simulink model "controllermodel"  (R2020a)
settings: Solver=FixedStepDiscrete  StartTime=0.0  StopTime=10.0  FixedStep=1/100  RelTol=1e-3
undefined symbols (not defined in the file): DiscIntNeverNeededParam
libraries: simulink_extras x3
settings Model: Creator=janik  LastModifiedBy=hopfj
settings OptimizationCC: DefaultParameterBehavior=Inlined  EnhancedBackFolding=on  PassReuseOutputArgsAs=Individual arguments  ZeroExternalMemoryAtStartup=off  ZeroInternalMemoryAtStartup=off  OptimizeBlockOrder=speed  DifferentSizesBufferReuse=on  OptimizationCustomize=off  EfficientTunableParamExpr=on
settings DebuggingCC: ParameterTunabilityLossMsg=error
settings SFSimCC: MATLABDynamicMemAlloc=off
settings RTWCC: SystemTargetFile=ert.tlc  GenCodeOnly=on  TemplateMakefile=ert_default_tmf  GenerateReport=on  Toolchain=Microsoft Visual C++ 2019 v16.0 | nmake (64-bit Windows)  LaunchReport=on  TargetLang=C++
settings CodeAppCC: ForceParamTrailComments=on  IgnoreCustomStorageClasses=off  OperatorAnnotations=on  SimulinkDataObjDesc=on  SFDataObjDesc=on  MATLABFcnDesc=on  InsertBlockDesc=on
settings ERTTargetCC: TargetLangStandard=C++03 (ISO)  GenerateSampleERTMain=on  CodeInterfacePackaging=C++ class  SupportVariableSizeSignals=on  InlinedParameterPlacement=NonHierarchical  RootIOFormat=Structure reference  ERTCustomFileTemplate=example_file_process.tlc

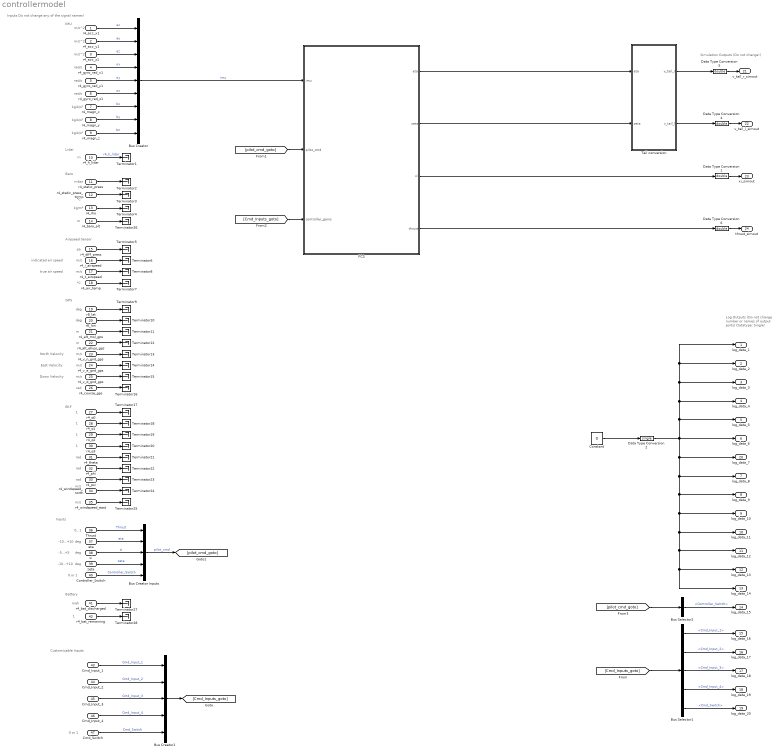
== system controllermodel ==
  note: Simulation Outputs
      | (Do not change!)
  note: m/s
  note: m/s
  note: Lidar
  note: kg/A/s²
  note: m/s
  note: m/s^2
  note: 1
  note: rad
  note: Down Velocity
  note: m
  note: m/s
  note: East Velocity
  note: kg/A/s²
  note: Inputs
      | Do not change any of the
      | signal names!
  note: m/s
  note: rad/s
  note: Airpseed Sensor
  note: Baro
  note: °C
  note: m/s
  note: Customizable Inputs
  note: kg/m³
  note: IMU
  note: pa
  note: 0...1
  note: m/s^2
  note: rad/s
  note: rad
  note: true air speed
  note: North Velocity
  note: mah
  note: m
  note: GPS
  note: kg/A/s²
  note: m/s
  note: rad/s
  note: mbar
  note: rad
  note: Inputs
  note: indicated air speed
  note: °C
  note: m
  note: m
  note: rad
  note: EKF
  note: Battery
  note: deg
  note: m/s^2
  note: deg
  note: Log Outputs
      | (Do not change
      | number or names
      | of output ports)
      | Datatype: Single!
  note: 0 or 1
  note: deg
  note: deg
  note: deg
  note: 1
  note: 1
  note: 1
  note: 1
  note: -10...+10
  note: -5...+5
  note: -10...+10
  note: 0 or 1
  r4_acc_x1 : Inport  OutDataTypeStr=single  Unit=m/s^2  PortDimensions=1  SampleTime=1/100  Interpolate=off
  r4_acc_y1 : Inport  Port=2  OutDataTypeStr=single  Unit=m/s^2  PortDimensions=1  SampleTime=1/100  Interpolate=off
  r4_acc_z1 : Inport  Port=3  OutDataTypeStr=single  Unit=m/s^2  PortDimensions=1  SampleTime=1/100  Interpolate=off
  r4_gyro_rad_x1 : Inport  Port=4  OutDataTypeStr=single  Unit=rad/s  PortDimensions=1  SampleTime=1/100  Interpolate=off
  r4_gyro_rad_y1 : Inport  Port=5  OutDataTypeStr=single  Unit=rad/s  PortDimensions=1  SampleTime=1/100  Interpolate=off
  r4_gyro_rad_z1 : Inport  Port=6  OutDataTypeStr=single  Unit=rad/s  PortDimensions=1  SampleTime=1/100  Interpolate=off  LockScale=on
  r4_magn_x : Inport  Port=7  OutDataTypeStr=single  Unit=kg/A/s^2  PortDimensions=1  SampleTime=1/100  Interpolate=off
  r4_magn_y : Inport  Port=8  OutDataTypeStr=single  Unit=kg/A/s^2  PortDimensions=1  SampleTime=1/100  Interpolate=off
  r4_magn_z : Inport  Port=9  OutDataTypeStr=single  Unit=kg/A/s^2  PortDimensions=1  SampleTime=1/100  Interpolate=off
  r4_h_lidar : Inport  Port=10  OutDataTypeStr=single  Unit=m  PortDimensions=1  SampleTime=1/100  Interpolate=off
  r4_static_press : Inport  Port=11  OutDataTypeStr=single  Unit=mbar  PortDimensions=1  SampleTime=1/100  Interpolate=off
  r4_static_press_temp : Inport  Port=12  OutDataTypeStr=single  Unit=°C  PortDimensions=1  SampleTime=1/100  Interpolate=off
  r4_rho : Inport  Port=13  OutDataTypeStr=single  Unit=kg/m^3  PortDimensions=1  SampleTime=1/100  Interpolate=off
  r4_baro_alt : Inport  Port=14  OutDataTypeStr=single  Unit=m  PortDimensions=1  SampleTime=1/100  Interpolate=off
  r4_diff_press : Inport  Port=15  OutDataTypeStr=single  Unit=Pa  PortDimensions=1  SampleTime=1/100  Interpolate=off
  r4_i_airspeed : Inport  Port=16  OutDataTypeStr=single  Unit=m/s  PortDimensions=1  SampleTime=1/100  Interpolate=off
  r4_t_airspeed : Inport  Port=17  OutDataTypeStr=single  Unit=m/s  PortDimensions=1  SampleTime=1/100  Interpolate=off
  r4_air_temp : Inport  Port=18  OutDataTypeStr=single  Unit=°C  PortDimensions=1  SampleTime=1/100  Interpolate=off
  r8_lat : Inport  Port=19  OutDataTypeStr=double  Unit=deg  PortDimensions=1  SampleTime=1/100  Interpolate=off
  r8_lon : Inport  Port=20  OutDataTypeStr=double  Unit=deg  PortDimensions=1  SampleTime=1/100  Interpolate=off
  r4_alt_msl_gps : Inport  Port=21  OutDataTypeStr=single  Unit=m  PortDimensions=1  SampleTime=1/100  Interpolate=off
  r4_alt_ellips_gps : Inport  Port=22  OutDataTypeStr=single  Unit=m  PortDimensions=1  SampleTime=1/100  Interpolate=off
  r4_v_n_gnd_gps : Inport  Port=23  OutDataTypeStr=single  Unit=m/s  PortDimensions=1  SampleTime=1/100  Interpolate=off
  r4_v_e_gnd_gps : Inport  Port=24  OutDataTypeStr=single  Unit=m/s  PortDimensions=1  SampleTime=1/100  Interpolate=off
  r4_v_d_gnd_gps : Inport  Port=25  OutDataTypeStr=single  Unit=m/s  PortDimensions=1  SampleTime=1/100  Interpolate=off
  r4_course_gps : Inport  Port=26  OutDataTypeStr=single  Unit=rad  PortDimensions=1  SampleTime=1/100  Interpolate=off
  r4_q0 : Inport  Port=27  OutMin=[-1]  OutMax=[1]  OutDataTypeStr=single  Unit=1  PortDimensions=1  SampleTime=1/100  Interpolate=off
  r4_q1 : Inport  Port=28  OutMin=[-1]  OutMax=[1]  OutDataTypeStr=single  Unit=1  PortDimensions=1  SampleTime=1/100  Interpolate=off
  r4_q2 : Inport  Port=29  OutMin=[-1]  OutMax=[1]  OutDataTypeStr=single  Unit=1  PortDimensions=1  SampleTime=1/100  Interpolate=off
  r4_q3 : Inport  Port=30  OutMin=[-1]  OutMax=[1]  OutDataTypeStr=single  Unit=one  PortDimensions=1  SampleTime=1/100  Interpolate=off
  r4_theta : Inport  Port=31  OutDataTypeStr=single  Unit=rad  PortDimensions=1  SampleTime=1/100  Interpolate=off
  r4_phi : Inport  Port=32  OutDataTypeStr=single  Unit=rad  PortDimensions=1  SampleTime=1/100  Interpolate=off
  r4_psi : Inport  Port=33  OutDataTypeStr=single  Unit=rad  PortDimensions=1  SampleTime=1/100  Interpolate=off
  r4_windspeed_north : Inport  Port=34  OutDataTypeStr=single  Unit=m/s  PortDimensions=1  SampleTime=1/100  Interpolate=off
  r4_windspeed_east : Inport  Port=35  OutDataTypeStr=single  Unit=m/s  PortDimensions=1  SampleTime=1/100  Interpolate=off
  Thrust : Inport  Port=36  OutDataTypeStr=single  PortDimensions=1  SampleTime=1/100  Interpolate=off
  eta : Inport  Port=37  OutDataTypeStr=single  Unit=deg  PortDimensions=1  SampleTime=1/100  Interpolate=off
  xi : Inport  Port=38  OutDataTypeStr=single  Unit=deg  PortDimensions=1  SampleTime=1/100  Interpolate=off
  zeta : Inport  Port=39  OutDataTypeStr=single  Unit=deg  PortDimensions=1  SampleTime=1/100  Interpolate=off
  Controller_Switch : Inport  Port=40  OutDataTypeStr=single  PortDimensions=1  SampleTime=1/100  Interpolate=off
  r4_bat_discharged : Inport  Port=41  OutDataTypeStr=single  Unit=mA*hr  PortDimensions=1  SampleTime=1/100  Interpolate=off
  r4_bat_remaining : Inport  Port=42  OutDataTypeStr=single  PortDimensions=1  SampleTime=1/100  Interpolate=off
  Cmd_Input_1 : Inport  Port=43  OutDataTypeStr=single  PortDimensions=1  SampleTime=1/100  Interpolate=off
  Cmd_Input_2 : Inport  Port=44  OutDataTypeStr=single  PortDimensions=1  SampleTime=1/100  Interpolate=off
  Cmd_Input_3 : Inport  Port=45  OutDataTypeStr=single  PortDimensions=1  SampleTime=1/100  Interpolate=off
  Cmd_Input_4 : Inport  Port=46  OutDataTypeStr=single  PortDimensions=1  SampleTime=1/100  Interpolate=off
  Cmd_Switch : Inport  Port=47  OutDataTypeStr=single  PortDimensions=1  SampleTime=1/100  Interpolate=off
  Bus Creator : BusCreator  Inputs=9
  Bus Creator Inputs : BusCreator  Inputs=5
  Bus Creator1 : BusCreator  Inputs=5
  Bus Selector1 : BusSelector  OutputSignals=Cmd_Input_1,Cmd_Input_2,Cmd_Input_3,Cmd_Input_4,Cmd_Switch
  Bus Selector2 : BusSelector  OutputSignals=Controller_Switch
  Constant : Constant  Value=0
  Data Type Conversion{1,4..6} (4 alike) : DataTypeConversion  OutDataTypeStr=double  RndMeth=Nearest
  Data Type Conversion2 : DataTypeConversion  OutDataTypeStr=single  RndMeth=Nearest
  FCS : Subsystem
  Tail conversion : Subsystem
  Terminator{1..28} (28 alike) : Terminator
  log_data_1 : Outport  OutDataTypeStr=single  SampleTime=1/100  VectorParamsAs1DForOutWhenUnconnected=off
  log_data_2 : Outport  Port=2  OutDataTypeStr=single  SampleTime=1/100  VectorParamsAs1DForOutWhenUnconnected=off
  log_data_3 : Outport  Port=3  OutDataTypeStr=single  SampleTime=1/100  VectorParamsAs1DForOutWhenUnconnected=off
  log_data_4 : Outport  Port=4  OutDataTypeStr=single  SampleTime=1/100  VectorParamsAs1DForOutWhenUnconnected=off
  log_data_5 : Outport  Port=5  OutDataTypeStr=single  SampleTime=1/100  VectorParamsAs1DForOutWhenUnconnected=off
  log_data_6 : Outport  Port=6  OutDataTypeStr=single  SampleTime=1/100  VectorParamsAs1DForOutWhenUnconnected=off
  log_data_8 : Outport  Port=7  OutDataTypeStr=single  SampleTime=1/100  VectorParamsAs1DForOutWhenUnconnected=off
  log_data_9 : Outport  Port=8  OutDataTypeStr=single  SampleTime=1/100  VectorParamsAs1DForOutWhenUnconnected=off
  log_data_10 : Outport  Port=9  OutDataTypeStr=single  SampleTime=1/100  VectorParamsAs1DForOutWhenUnconnected=off
  log_data_11 : Outport  Port=10  OutDataTypeStr=single  SampleTime=1/100  VectorParamsAs1DForOutWhenUnconnected=off
  log_data_12 : Outport  Port=11  OutDataTypeStr=single  SampleTime=1/100  VectorParamsAs1DForOutWhenUnconnected=off
  log_data_13 : Outport  Port=12  OutDataTypeStr=single  SampleTime=1/100  VectorParamsAs1DForOutWhenUnconnected=off
  log_data_14 : Outport  Port=13  OutDataTypeStr=single  SampleTime=1/100  VectorParamsAs1DForOutWhenUnconnected=off
  log_data_15 : Outport  Port=14  OutDataTypeStr=single  SampleTime=1/100  VectorParamsAs1DForOutWhenUnconnected=off
  log_data_16 : Outport  Port=15  OutDataTypeStr=single  SampleTime=1/100  VectorParamsAs1DForOutWhenUnconnected=off
  log_data_17 : Outport  Port=16  OutDataTypeStr=single  SampleTime=1/100  VectorParamsAs1DForOutWhenUnconnected=off
  log_data_18 : Outport  Port=17  OutDataTypeStr=single  SampleTime=1/100  VectorParamsAs1DForOutWhenUnconnected=off
  log_data_19 : Outport  Port=18  OutDataTypeStr=single  SampleTime=1/100  VectorParamsAs1DForOutWhenUnconnected=off
  log_data_20 : Outport  Port=19  OutDataTypeStr=single  SampleTime=1/100  VectorParamsAs1DForOutWhenUnconnected=off
  log_data_7 : Outport  Port=20  OutDataTypeStr=single  SampleTime=1/100  VectorParamsAs1DForOutWhenUnconnected=off
  v_tail_r_simout : Outport  Port=21  OutDataTypeStr=double  Unit=rad  SampleTime=1/100  VectorParamsAs1DForOutWhenUnconnected=off
  v_tail_l_simout : Outport  Port=22  OutDataTypeStr=double  Unit=rad  SampleTime=1/100  VectorParamsAs1DForOutWhenUnconnected=off
  xi_simout : Outport  Port=23  OutDataTypeStr=double  Unit=rad  SampleTime=1/100  VectorParamsAs1DForOutWhenUnconnected=off
  thrust_simout : Outport  Port=24  OutDataTypeStr=double  SampleTime=1/100  VectorParamsAs1DForOutWhenUnconnected=off
  wires:
  r4_phi/1 -> Terminator22/1
  Controller_Switch/1 -> Bus Creator Inputs/5  "Controller_Switch"
  r4_h_lidar/1 -> Terminator1/1  "r4_h_lidar"
  r4_gyro_rad_y1/1 -> Bus Creator/5  "oy"
  r4_rho/1 -> Terminator4/1
  FCS/1(eta) -> Tail conversion/1(eta)
  r4_static_press_temp/1 -> Terminator3/1
  r4_air_temp/1 -> Terminator7/1
  r4_alt_msl_gps/1 -> Terminator11/1
  r4_diff_press/1 -> Terminator5/1
  r4_acc_z1/1 -> Bus Creator/3  "az"
  xi/1 -> Bus Creator Inputs/3  "xi"
  Thrust/1 -> Bus Creator Inputs/1  "Thrust"
  r4_course_gps/1 -> Terminator16/1
  r4_q0/1 -> Terminator17/1
  Tail conversion/1(v_tail_r) -> Data Type Conversion5/1
  r4_v_n_gnd_gps/1 -> Terminator13/1
  Tail conversion/2(v_tail_l) -> Data Type Conversion4/1
  r4_magn_x/1 -> Bus Creator/7  "bx"
  FCS/3(xi) -> Data Type Conversion1/1
  r4_acc_y1/1 -> Bus Creator/2  "ay"
  r4_psi/1 -> Terminator23/1
  r4_v_e_gnd_gps/1 -> Terminator14/1
  r4_gyro_rad_x1/1 -> Bus Creator/4  "ox"
  r4_bat_discharged/1 -> Terminator27/1
  r4_baro_alt/1 -> Terminator26/1
  FCS/4(thrust) -> Data Type Conversion6/1
  r4_v_d_gnd_gps/1 -> Terminator15/1
  r4_q2/1 -> Terminator19/1
  r4_static_press/1 -> Terminator2/1
  Cmd_Input_1/1 -> Bus Creator1/1  "Cmd_Input_1"
  r4_gyro_rad_z1/1 -> Bus Creator/6  "oz"
  zeta/1 -> Bus Creator Inputs/4  "zeta"
  r4_magn_z/1 -> Bus Creator/9  "bz"
  r8_lat/1 -> Terminator9/1
  r8_lon/1 -> Terminator10/1
  r4_t_airspeed/1 -> Terminator8/1
  r4_magn_y/1 -> Bus Creator/8  "by"
  Cmd_Input_2/1 -> Bus Creator1/2  "Cmd_Input_2"
  r4_alt_ellips_gps/1 -> Terminator12/1
  r4_windspeed_east/1 -> Terminator25/1
  r4_windspeed_north/1 -> Terminator24/1
  Cmd_Input_4/1 -> Bus Creator1/4  "Cmd_Input_4"
  FCS/2(zeta) -> Tail conversion/2(zeta)
  eta/1 -> Bus Creator Inputs/2  "eta"
  Cmd_Input_3/1 -> Bus Creator1/3  "Cmd_Input_3"
  r4_q1/1 -> Terminator18/1
  r4_q3/1 -> Terminator20/1
  r4_bat_remaining/1 -> Terminator28/1
  r4_i_airspeed/1 -> Terminator6/1
  r4_acc_x1/1 -> Bus Creator/1  "ax"
  Constant/1 -> Data Type Conversion2/1
  Bus Creator/1 -> FCS/1(imu)  "imu"
  r4_theta/1 -> Terminator21/1
  Bus Creator1/1 -> [Cmd_Inputs_goto]
  [Cmd_Inputs_goto] -> Bus Selector1/1
  Bus Creator Inputs/1 -> [pilot_cmd_goto]  "pilot_cmd"
  Data Type Conversion1/1 -> xi_simout/1
  Data Type Conversion5/1 -> v_tail_r_simout/1
  Data Type Conversion4/1 -> v_tail_l_simout/1
  Data Type Conversion6/1 -> thrust_simout/1
  [pilot_cmd_goto] -> FCS/2(pilot_cmd)
  [Cmd_Inputs_goto] -> FCS/3(controller_gains)
  Data Type Conversion2/1 -> log_data_1/1, log_data_2/1, log_data_3/1, log_data_4/1, log_data_5/1, log_data_6/1, log_data_7/1, log_data_8/1, log_data_9/1, log_data_10/1, log_data_11/1, log_data_14/1, log_data_13/1, log_data_12/1
  Bus Selector1/2 -> log_data_17/1  "<Cmd_Input_2>"
  Bus Selector1/3 -> log_data_18/1  "<Cmd_Input_3>"
  Bus Selector1/4 -> log_data_19/1  "<Cmd_Input_4>"
  Bus Selector1/5 -> log_data_20/1  "<Cmd_Switch>"
  [pilot_cmd_goto] -> Bus Selector2/1
  Bus Selector2/1 -> log_data_15/1  "<Controller_Switch>"
  Cmd_Switch/1 -> Bus Creator1/5  "Cmd_Switch"
  Bus Selector1/1 -> log_data_16/1  "<Cmd_Input_1>"

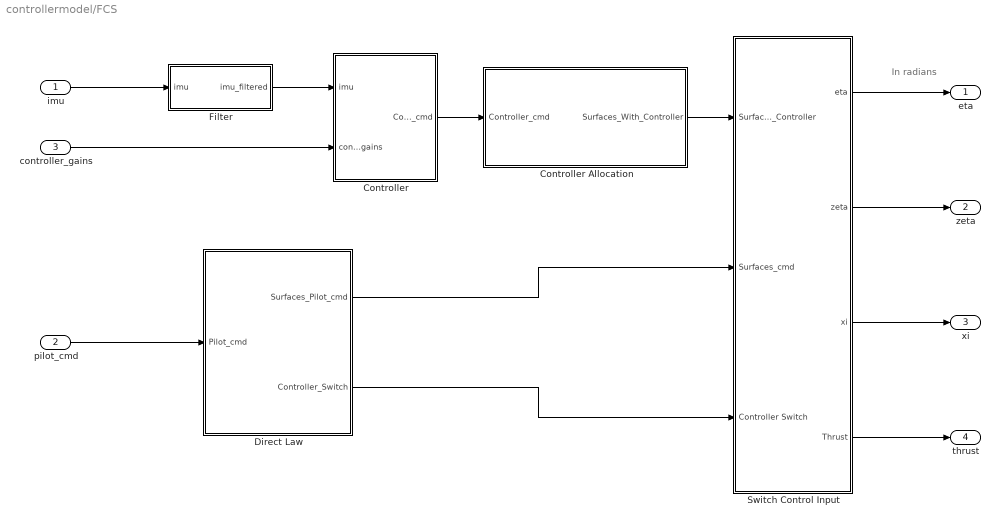
== system controllermodel/FCS ==
  note: In radians
  imu : Inport
  pilot_cmd : Inport  Port=2
  controller_gains : Inport  Port=3
  Controller : Subsystem
  Controller Allocation : Subsystem
  Direct Law : Subsystem
  Filter : Subsystem
  Switch Control Input : Subsystem
  eta : Outport  Unit=rad
  zeta : Outport  Port=2  Unit=rad
  xi : Outport  Port=3  Unit=rad
  thrust : Outport  Port=4  Unit=rad
  wires:
  Controller Allocation/1(Surfaces_With_Controller) -> Switch Control Input/1(Surfaces_With_Controller)
  pilot_cmd/1 -> Direct Law/1(Pilot_cmd)
  imu/1 -> Filter/1(imu)
  Switch Control Input/4(Thrust) -> thrust/1
  Switch Control Input/2(zeta) -> zeta/1
  Switch Control Input/1(eta) -> eta/1
  Switch Control Input/3(xi) -> xi/1
  Filter/1(imu_filtered) -> Controller/1(imu)
  Direct Law/2(Controller_Switch) -> Switch Control Input/3(Controller Switch)
  controller_gains/1 -> Controller/2(controller_gains)
  Direct Law/1(Surfaces_Pilot_cmd) -> Switch Control Input/2(Surfaces_cmd)
  Controller/1(Controller_cmd) -> Controller Allocation/1(Controller_cmd)

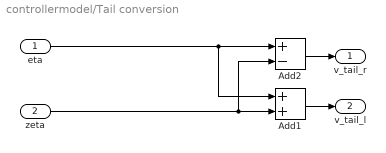
== system controllermodel/Tail conversion ==
  eta : Inport  Unit=rad
  zeta : Inport  Port=2  Unit=rad
  Add1 : Sum  OutDataTypeStr=double
  Add2 : Sum  Inputs=+-  InputSameDT=on  OutDataTypeStr=double
  v_tail_r : Outport  Unit=rad
  v_tail_l : Outport  Port=2  Unit=rad
  wires:
  Add1/1 -> v_tail_l/1
  Add2/1 -> v_tail_r/1
  zeta/1 -> Add2/2, Add1/2
  eta/1 -> Add2/1, Add1/1

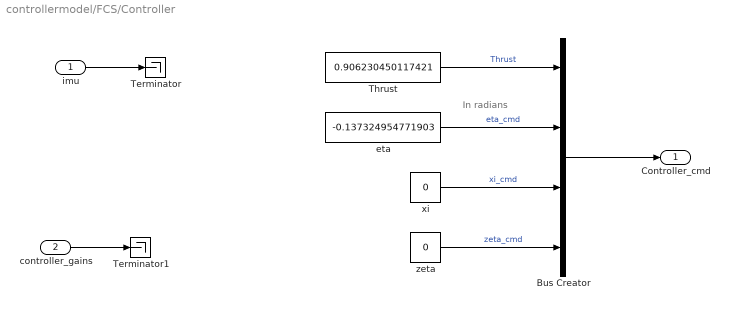
== system controllermodel/FCS/Controller ==
  note: In radians
  imu : Inport
  controller_gains : Inport  Port=2
  Bus Creator : BusCreator  Inputs=4
  Terminator : Terminator
  Terminator1 : Terminator
  Thrust : Constant  Value=0.906230450117421
  eta : Constant  Value=-0.137324954771903
  xi : Constant  Value=0
  zeta : Constant  Value=0
  Controller_cmd : Outport
  wires:
  Bus Creator/1 -> Controller_cmd/1
  imu/1 -> Terminator/1
  controller_gains/1 -> Terminator1/1
  Thrust/1 -> Bus Creator/1  "Thrust"
  eta/1 -> Bus Creator/2  "eta_cmd"
  xi/1 -> Bus Creator/3  "xi_cmd"
  zeta/1 -> Bus Creator/4  "zeta_cmd"

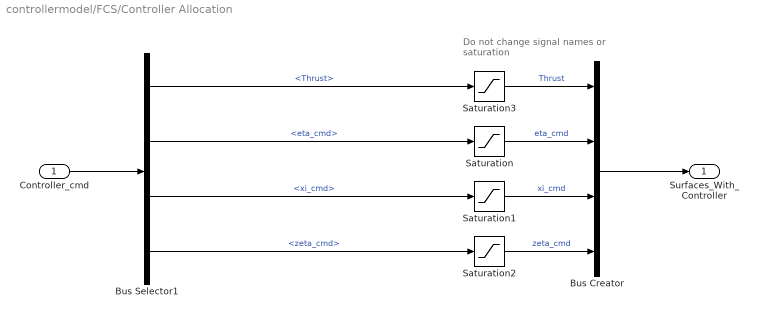
== system controllermodel/FCS/Controller Allocation ==
  note: Do not change signal names
      | or saturation
  Controller_cmd : Inport
  Bus Creator : BusCreator  Inputs=4
  Bus Selector1 : BusSelector  OutputSignals=Thrust,eta_cmd,xi_cmd,zeta_cmd
  Saturation : Saturate  UpperLimit=deg2rad(10)  LowerLimit=deg2rad(-20)
  Saturation1 : Saturate  UpperLimit=deg2rad(5)  LowerLimit=deg2rad(-5)
  Saturation2 : Saturate  UpperLimit=deg2rad(10)  LowerLimit=deg2rad(-10)
  Saturation3 : Saturate  UpperLimit=1  LowerLimit=0
  Surfaces_With_Controller : Outport
  wires:
  Bus Creator/1 -> Surfaces_With_Controller/1
  Controller_cmd/1 -> Bus Selector1/1
  Bus Selector1/4 -> Saturation2/1  "<zeta_cmd>"
  Bus Selector1/3 -> Saturation1/1  "<xi_cmd>"
  Bus Selector1/2 -> Saturation/1  "<eta_cmd>"
  Bus Selector1/1 -> Saturation3/1  "<Thrust>"
  Saturation/1 -> Bus Creator/2  "eta_cmd"
  Saturation1/1 -> Bus Creator/3  "xi_cmd"
  Saturation2/1 -> Bus Creator/4  "zeta_cmd"
  Saturation3/1 -> Bus Creator/1  "Thrust"

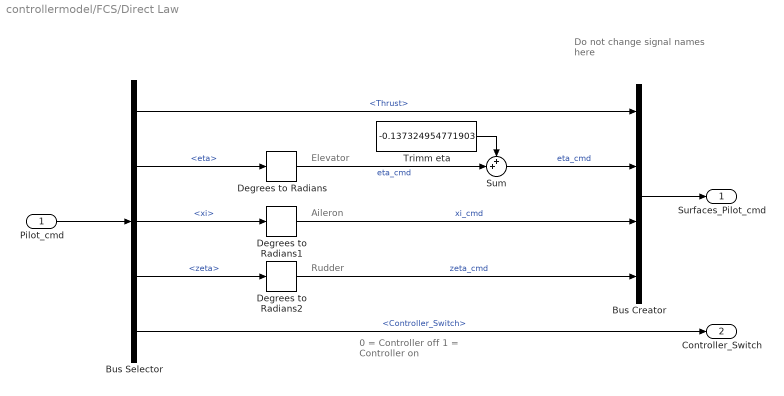
== system controllermodel/FCS/Direct Law ==
  note: Elevator
  note: 0 = Controller off
      | 1 = Controller on
  note: Do not change
      | signal names
      | here
  note: Aileron
  note: Rudder
  Pilot_cmd : Inport
  Bus Creator : BusCreator  Inputs=4
  Bus Selector : BusSelector  OutputSignals=Thrust,eta,xi,zeta,Controller_Switch
  Degrees to Radians : simulink_extras/Transformations/Degrees to Radians
  Degrees to Radians1 : simulink_extras/Transformations/Degrees to Radians
  Degrees to Radians2 : simulink_extras/Transformations/Degrees to Radians
  Sum : Sum  Inputs=++|
  Trimm eta : Constant  Description=trim thrust  Value=-0.137324954771903  OutDataTypeStr=double
  Surfaces_Pilot_cmd : Outport
  Controller_Switch : Outport  Port=2
  wires:
  Pilot_cmd/1 -> Bus Selector/1
  Bus Selector/1 -> Bus Creator/1  "<Thrust>"
  Bus Selector/2 -> Degrees to Radians/1  "<eta>"
  Bus Selector/4 -> Degrees to Radians2/1  "<zeta>"
  Bus Selector/3 -> Degrees to Radians1/1  "<xi>"
  Bus Selector/5 -> Controller_Switch/1  "<Controller_Switch>"
  Bus Creator/1 -> Surfaces_Pilot_cmd/1
  Sum/1 -> Bus Creator/2  "eta_cmd"
  Degrees to Radians1/1 -> Bus Creator/3  "xi_cmd"
  Degrees to Radians2/1 -> Bus Creator/4  "zeta_cmd"
  Degrees to Radians/1 -> Sum/2  "eta_cmd"
  Trimm eta/1 -> Sum/1

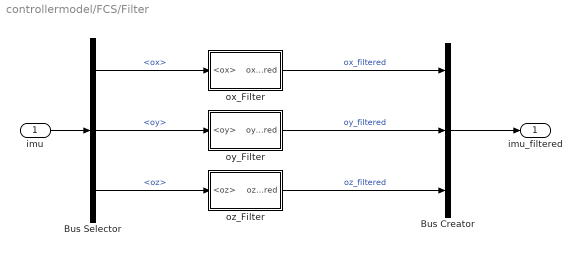
== system controllermodel/FCS/Filter ==
  imu : Inport
  Bus Creator : BusCreator  Inputs=3
  Bus Selector : BusSelector  OutputSignals=ox,oy,oz
  ox_Filter : Subsystem
  oy_Filter : Subsystem
  oz_Filter : Subsystem
  imu_filtered : Outport
  wires:
  imu/1 -> Bus Selector/1
  Bus Selector/1 -> ox_Filter/1(<ox>)  "<ox>"
  ox_Filter/1(ox_filtered) -> Bus Creator/1  "ox_filtered"
  Bus Selector/2 -> oy_Filter/1(<oy>)  "<oy>"
  oy_Filter/1(oy_filtered) -> Bus Creator/2  "oy_filtered"
  Bus Selector/3 -> oz_Filter/1(<oz>)  "<oz>"
  oz_Filter/1(oz_filtered) -> Bus Creator/3  "oz_filtered"
  Bus Creator/1 -> imu_filtered/1

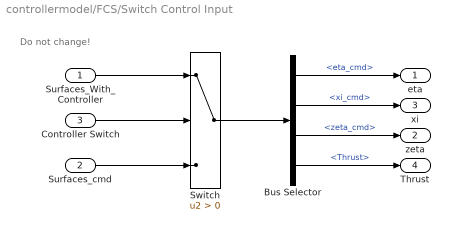
== system controllermodel/FCS/Switch Control Input ==
  note: Do not change!
  Surfaces_With_Controller : Inport
  Surfaces_cmd : Inport  Port=2
  Controller Switch : Inport  Port=3
  Bus Selector : BusSelector  OutputSignals=eta_cmd,xi_cmd,zeta_cmd,Thrust
  Switch : Switch  Criteria=u2 > Threshold
  eta : Outport
  zeta : Outport  Port=2
  xi : Outport  Port=3
  Thrust : Outport  Port=4
  wires:
  Surfaces_With_Controller/1 -> Switch/1
  Controller Switch/1 -> Switch/2
  Surfaces_cmd/1 -> Switch/3
  Switch/1 -> Bus Selector/1
  Bus Selector/1 -> eta/1  "<eta_cmd>"
  Bus Selector/2 -> xi/1  "<xi_cmd>"
  Bus Selector/3 -> zeta/1  "<zeta_cmd>"
  Bus Selector/4 -> Thrust/1  "<Thrust>"

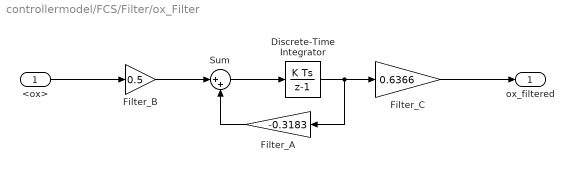
== system controllermodel/FCS/Filter/ox_Filter ==
  <ox> : Inport
  Discrete-Time Integrator : DiscreteIntegrator  SampleTime=-1  ICPrevOutput=DiscIntNeverNeededParam  ICPrevScaledInput=DiscIntNeverNeededParam
  Filter_A : Gain  Gain=-0.3183
  Filter_B : Gain  Gain=0.5
  Filter_C : Gain  Gain=0.6366
  Sum : Sum  Inputs=|++
  ox_filtered : Outport
  wires:
  <ox>/1 -> Filter_B/1
  Filter_C/1 -> ox_filtered/1
  Filter_B/1 -> Sum/1
  Discrete-Time Integrator/1 -> Filter_A/1, Filter_C/1
  Filter_A/1 -> Sum/2
  Sum/1 -> Discrete-Time Integrator/1

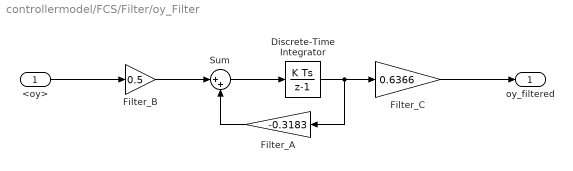
== system controllermodel/FCS/Filter/oy_Filter ==
  <oy> : Inport
  Discrete-Time Integrator : DiscreteIntegrator  SampleTime=-1  ICPrevOutput=DiscIntNeverNeededParam  ICPrevScaledInput=DiscIntNeverNeededParam
  Filter_A : Gain  Gain=-0.3183
  Filter_B : Gain  Gain=0.5
  Filter_C : Gain  Gain=0.6366
  Sum : Sum  Inputs=|++
  oy_filtered : Outport
  wires:
  <oy>/1 -> Filter_B/1
  Filter_C/1 -> oy_filtered/1
  Filter_B/1 -> Sum/1
  Discrete-Time Integrator/1 -> Filter_A/1, Filter_C/1
  Filter_A/1 -> Sum/2
  Sum/1 -> Discrete-Time Integrator/1

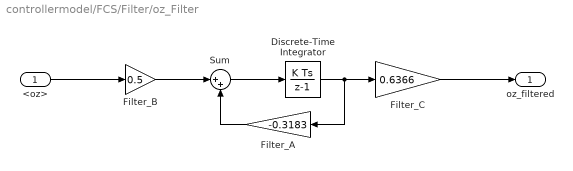
== system controllermodel/FCS/Filter/oz_Filter ==
  <oz> : Inport
  Discrete-Time Integrator : DiscreteIntegrator  SampleTime=-1  ICPrevOutput=DiscIntNeverNeededParam  ICPrevScaledInput=DiscIntNeverNeededParam
  Filter_A : Gain  Gain=-0.3183
  Filter_B : Gain  Gain=0.5
  Filter_C : Gain  Gain=0.6366
  Sum : Sum  Inputs=|++
  oz_filtered : Outport
  wires:
  Sum/1 -> Discrete-Time Integrator/1
  Filter_A/1 -> Sum/2
  Discrete-Time Integrator/1 -> Filter_C/1, Filter_A/1
  Filter_B/1 -> Sum/1
  Filter_C/1 -> oz_filtered/1
  <oz>/1 -> Filter_B/1
